simulink model "HaroldPractice"  (R2025b)
settings: Solver=VariableStepAuto  StartTime=0.0  StopTime=10.0  RelTol=1e-3
undefined symbols (not defined in the file): ChargingWire, DataIN, DataOUT, DisplayLink, OutputWire
settings Model: Creator=jakeo  LastModifiedBy=jakeo

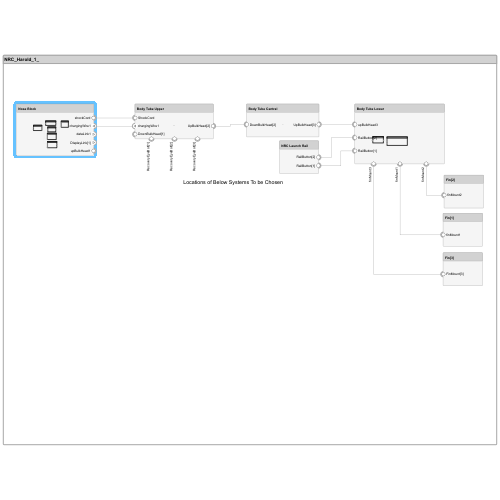
[thumbnail: Simulink's stored preview of the top-level diagram]
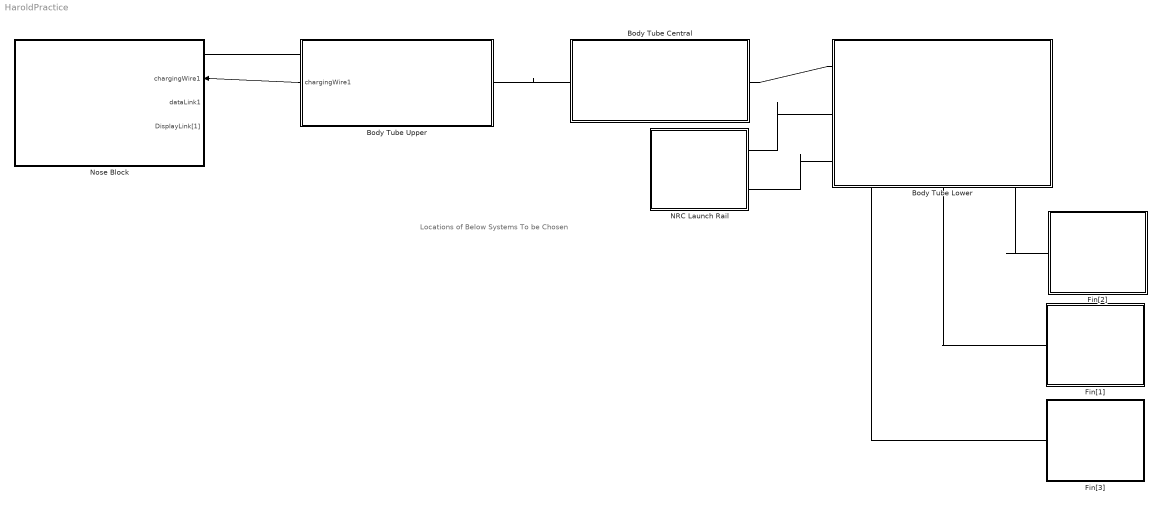
== system HaroldPractice ==
  note: Locations of Below Systems To be Chosen
  Body Tube Central : Subsystem
      settings: PortSchema="{\"entries\":[{\"content\":{\"headerSize\":26,\"margin\":15,\"minimumSpacing\":25,\"sides\":[{\"content\":{\"connectorIds\":[\"LConn1\"]},\"type\":\"ConnectorPlacement.EquallySpacedRectSide\",\"uuid\":\"03e957df-4bae-46ab-9d0d-48f80a496ac5\"},{\"content\":{\"connectorIds\":[\"RConn1\"],\"side\":\"RIGHT\"},\"type\":\"ConnectorPlacement.EquallySpacedRectSide\",\"uuid\":\"d2433d43-ba0e-4345-8a8e-99b57dcef125\"},{\"content\":{\"side\":\"TOP\"},\"type\":\"ConnectorPlacement.EquallySpacedRectSide\",\"uuid\":\"84844adf-0e3d-439c-a28c-7cf27e8d243a\"}]},\"type\":\"ConnectorPlacement.EquallySpacedConnector\",\"uuid\":\"9b26577b-50b2-4983-8f3c-4df87f23ba49\"}],\"packageUris\":[\"http://schema.mathworks.com/mf0/Connector/R2020b\"],\"version\":\"1.0\"}"
  Body Tube Lower : Subsystem
      settings: PortSchema="{\"entries\":[{\"content\":{\"headerSize\":26,\"margin\":15,\"minimumSpacing\":25,\"sides\":[{\"content\":{\"connectorIds\":[\"LConn1\",\"LConn4\",\"LConn5\"]},\"type\":\"ConnectorPlacement.EquallySpacedRectSide\",\"uuid\":\"03e957df-4bae-46ab-9d0d-48f80a496ac5\"},{\"content\":{\"side\":\"RIGHT\"},\"type\":\"ConnectorPlacement.EquallySpacedRectSide\",\"uuid\":\"d2433d43-ba0e-4345-8a8e-99b57dcef125\"},{\"content\":{\"side\":\"TOP\"},\"type\":\"ConnectorPlacement.EquallySpacedRectSide\",\"uuid\":\"84844adf-0e3d-439c-a28c-7cf27e8d243a\"},{\"content\":{\"connectorIds\":[\"LConn3\",\"LConn6\",\"LConn2\"],\"side\":\"BOTTOM\"},\"type\":\"ConnectorPlacement.EquallySpacedRectSide\",\"uuid\":\"9b3a5652-69bd-4b6e-9b29-131929afca7c\"}]},\"type\":\"ConnectorPlacement.EquallySpacedConnector\",\"uuid\":\"9b26577b-50b2-4983-8f3c-4df87f23ba49\"}],\"packageUris\":[\"http://schema.mathworks.com/mf0/Connector/R2020b\"],\"version\":\"1.0\"}"
  Body Tube Upper : Subsystem
      settings: PortSchema="{\"entries\":[{\"content\":{\"headerSize\":26,\"margin\":15,\"minimumSpacing\":25,\"sides\":[{\"content\":{\"connectorIds\":[\"LConn1\",\"Out1\",\"LConn2\"]},\"type\":\"ConnectorPlacement.EquallySpacedRectSide\",\"uuid\":\"03e957df-4bae-46ab-9d0d-48f80a496ac5\"},{\"content\":{\"connectorIds\":[\"RConn1\"],\"side\":\"RIGHT\"},\"type\":\"ConnectorPlacement.EquallySpacedRectSide\",\"uuid\":\"d2433d43-ba0e-4345-8a8e-99b57dcef125\"},{\"content\":{\"side\":\"TOP\"},\"type\":\"ConnectorPlacement.EquallySpacedRectSide\",\"uuid\":\"84844adf-0e3d-439c-a28c-7cf27e8d243a\"},{\"content\":{\"connectorIds\":[\"RConn2\",\"RConn3\",\"RConn4\"],\"side\":\"BOTTOM\"},\"type\":\"ConnectorPlacement.EquallySpacedRectSide\",\"uuid\":\"7d79bddd-aaf5-48a9-85da-385393746c36\"}]},\"type\":\"ConnectorPlacement.EquallySpacedConnector\",\"uuid\":\"9b26577b-50b2-4983-8f3c-4df87f23ba49\"}],\"packageUris\":[\"http://schema.mathworks.com/mf0/Connector/R2020b\"],\"version\":\"1.0\"}"
  Fin[1] : Subsystem
      settings: PortSchema="{\"entries\":[{\"content\":{\"headerSize\":26,\"margin\":15,\"minimumSpacing\":25,\"sides\":[{\"content\":{\"connectorIds\":[\"LConn1\"]},\"type\":\"ConnectorPlacement.EquallySpacedRectSide\",\"uuid\":\"03e957df-4bae-46ab-9d0d-48f80a496ac5\"},{\"content\":{\"side\":\"RIGHT\"},\"type\":\"ConnectorPlacement.EquallySpacedRectSide\",\"uuid\":\"d2433d43-ba0e-4345-8a8e-99b57dcef125\"},{\"content\":{\"side\":\"TOP\"},\"type\":\"ConnectorPlacement.EquallySpacedRectSide\",\"uuid\":\"84844adf-0e3d-439c-a28c-7cf27e8d243a\"}]},\"type\":\"ConnectorPlacement.EquallySpacedConnector\",\"uuid\":\"9b26577b-50b2-4983-8f3c-4df87f23ba49\"}],\"packageUris\":[\"http://schema.mathworks.com/mf0/Connector/R2020b\"],\"version\":\"1.0\"}"
  Fin[2] : Subsystem
      settings: PortSchema="{\"entries\":[{\"content\":{\"headerSize\":26,\"margin\":15,\"minimumSpacing\":25,\"sides\":[{\"content\":{\"connectorIds\":[\"LConn1\"]},\"type\":\"ConnectorPlacement.EquallySpacedRectSide\",\"uuid\":\"03e957df-4bae-46ab-9d0d-48f80a496ac5\"},{\"content\":{\"side\":\"RIGHT\"},\"type\":\"ConnectorPlacement.EquallySpacedRectSide\",\"uuid\":\"d2433d43-ba0e-4345-8a8e-99b57dcef125\"},{\"content\":{\"side\":\"TOP\"},\"type\":\"ConnectorPlacement.EquallySpacedRectSide\",\"uuid\":\"84844adf-0e3d-439c-a28c-7cf27e8d243a\"}]},\"type\":\"ConnectorPlacement.EquallySpacedConnector\",\"uuid\":\"9b26577b-50b2-4983-8f3c-4df87f23ba49\"}],\"packageUris\":[\"http://schema.mathworks.com/mf0/Connector/R2020b\"],\"version\":\"1.0\"}"
  Fin[3] : Subsystem
      settings: PortSchema="{\"entries\":[{\"content\":{\"headerSize\":26,\"margin\":15,\"minimumSpacing\":25,\"sides\":[{\"content\":{\"connectorIds\":[\"LConn1\"]},\"type\":\"ConnectorPlacement.EquallySpacedRectSide\",\"uuid\":\"03e957df-4bae-46ab-9d0d-48f80a496ac5\"},{\"content\":{\"side\":\"RIGHT\"},\"type\":\"ConnectorPlacement.EquallySpacedRectSide\",\"uuid\":\"d2433d43-ba0e-4345-8a8e-99b57dcef125\"},{\"content\":{\"side\":\"TOP\"},\"type\":\"ConnectorPlacement.EquallySpacedRectSide\",\"uuid\":\"84844adf-0e3d-439c-a28c-7cf27e8d243a\"}]},\"type\":\"ConnectorPlacement.EquallySpacedConnector\",\"uuid\":\"9b26577b-50b2-4983-8f3c-4df87f23ba49\"}],\"packageUris\":[\"http://schema.mathworks.com/mf0/Connector/R2020b\"],\"version\":\"1.0\"}"
  NRC Launch Rail : Subsystem
      settings: PortSchema="{\"entries\":[{\"content\":{\"headerSize\":26,\"margin\":15,\"minimumSpacing\":25,\"sides\":[{\"content\":{},\"type\":\"ConnectorPlacement.EquallySpacedRectSide\",\"uuid\":\"6f4db608-f49c-4d1a-85cc-b66ec62c2f96\"},{\"content\":{\"connectorIds\":[\"RConn2\",\"RConn1\"],\"side\":\"RIGHT\"},\"type\":\"ConnectorPlacement.EquallySpacedRectSide\",\"uuid\":\"3e275c67-1c5c-46cd-973f-75adcfca9e5d\"},{\"content\":{\"side\":\"TOP\"},\"type\":\"ConnectorPlacement.EquallySpacedRectSide\",\"uuid\":\"88fdcd36-c2bf-423f-a1bd-8e2b1c2ac438\"}]},\"type\":\"ConnectorPlacement.EquallySpacedConnector\",\"uuid\":\"596a3d77-8add-49e5-be48-e23e6a2b115a\"}],\"packageUris\":[\"http://schema.mathworks.com/mf0/Connector/R2020b\"],\"version\":\"1.0\"}"
  Nose Block : Subsystem
      settings: PortSchema="{\"entries\":[{\"content\":{\"headerSize\":26,\"margin\":15,\"minimumSpacing\":25,\"sides\":[{\"content\":{},\"type\":\"ConnectorPlacement.EquallySpacedRectSide\",\"uuid\":\"03e957df-4bae-46ab-9d0d-48f80a496ac5\"},{\"content\":{\"connectorIds\":[\"LConn1\",\"In1\",\"Out1\",\"Out2\",\"RConn1\"],\"side\":\"RIGHT\"},\"type\":\"ConnectorPlacement.EquallySpacedRectSide\",\"uuid\":\"d2433d43-ba0e-4345-8a8e-99b57dcef125\"},{\"content\":{\"side\":\"TOP\"},\"type\":\"ConnectorPlacement.EquallySpacedRectSide\",\"uuid\":\"84844adf-0e3d-439c-a28c-7cf27e8d243a\"}]},\"type\":\"ConnectorPlacement.EquallySpacedConnector\",\"uuid\":\"9b26577b-50b2-4983-8f3c-4df87f23ba49\"}],\"packageUris\":[\"http://schema.mathworks.com/mf0/Connector/R2020b\"],\"version\":\"1.0\"}"
  wires:
  Body Tube Upper/1(chargingWire1) -> Nose Block/1(chargingWire1)
  connections:
  Nose Block/LConn1 -- Body Tube Upper/LConn1
  Body Tube Upper/RConn1 -- Body Tube Central/LConn1
  Body Tube Central/RConn1 -- Body Tube Lower/LConn1
  Fin[2]/LConn1 -- Body Tube Lower/LConn2
  Fin[1]/LConn1 -- Body Tube Lower/LConn6
  Fin[3]/LConn1 -- Body Tube Lower/LConn3
  NRC Launch Rail/RConn1 -- Body Tube Lower/LConn5
  NRC Launch Rail/RConn2 -- Body Tube Lower/LConn4

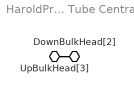
== system HaroldPractice/Body Tube Central ==
  DownBulkHead[2] : PMIOPort  Side=Left
  UpBulkHead[3] : PMIOPort  Port=2  Side=Right
  connections:
  UpBulkHead[3]/RConn1 -- DownBulkHead[2]/RConn1

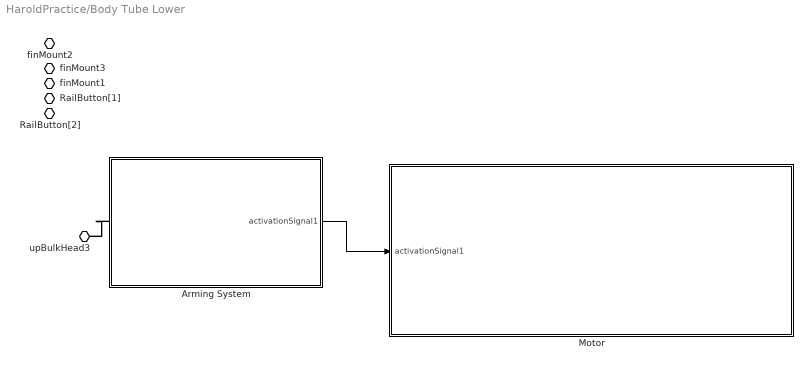
== system HaroldPractice/Body Tube Lower ==
  Arming System : Subsystem
      settings: PortSchema="{\"entries\":[{\"content\":{\"headerSize\":26,\"margin\":15,\"minimumSpacing\":25,\"sides\":[{\"content\":{\"connectorIds\":[\"LConn1\"]},\"type\":\"ConnectorPlacement.EquallySpacedRectSide\",\"uuid\":\"6f4db608-f49c-4d1a-85cc-b66ec62c2f96\"},{\"content\":{\"connectorIds\":[\"Out1\"],\"side\":\"RIGHT\"},\"type\":\"ConnectorPlacement.EquallySpacedRectSide\",\"uuid\":\"3e275c67-1c5c-46cd-973f-75adcfca9e5d\"},{\"content\":{\"side\":\"TOP\"},\"type\":\"ConnectorPlacement.EquallySpacedRectSide\",\"uuid\":\"88fdcd36-c2bf-423f-a1bd-8e2b1c2ac438\"}]},\"type\":\"ConnectorPlacement.EquallySpacedConnector\",\"uuid\":\"596a3d77-8add-49e5-be48-e23e6a2b115a\"}],\"packageUris\":[\"http://schema.mathworks.com/mf0/Connector/R2020b\"],\"version\":\"1.0\"}"
  Motor : Subsystem
      settings: PortSchema="{\"entries\":[{\"content\":{\"headerSize\":26,\"margin\":15,\"minimumSpacing\":25,\"sides\":[{\"content\":{\"connectorIds\":[\"LConn1\",\"In1\",\"LConn2\"]},\"type\":\"ConnectorPlacement.EquallySpacedRectSide\",\"uuid\":\"03e957df-4bae-46ab-9d0d-48f80a496ac5\"},{\"content\":{\"side\":\"RIGHT\"},\"type\":\"ConnectorPlacement.EquallySpacedRectSide\",\"uuid\":\"d2433d43-ba0e-4345-8a8e-99b57dcef125\"},{\"content\":{\"side\":\"TOP\"},\"type\":\"ConnectorPlacement.EquallySpacedRectSide\",\"uuid\":\"84844adf-0e3d-439c-a28c-7cf27e8d243a\"}]},\"type\":\"ConnectorPlacement.EquallySpacedConnector\",\"uuid\":\"9b26577b-50b2-4983-8f3c-4df87f23ba49\"}],\"packageUris\":[\"http://schema.mathworks.com/mf0/Connector/R2020b\"],\"version\":\"1.0\"}"
  upBulkHead3 : PMIOPort  Side=Left
  finMount2 : PMIOPort  Port=2  Side=Left
  finMount3 : PMIOPort  Port=3  Side=Left
  RailButton[2] : PMIOPort  Port=4  Side=Left
  RailButton[1] : PMIOPort  Port=5  Side=Left
  finMount1 : PMIOPort  Port=6  Side=Left
  wires:
  Arming System/1(activationSignal1) -> Motor/1(activationSignal1)
  connections:
  Arming System/LConn1 -- upBulkHead3/RConn1

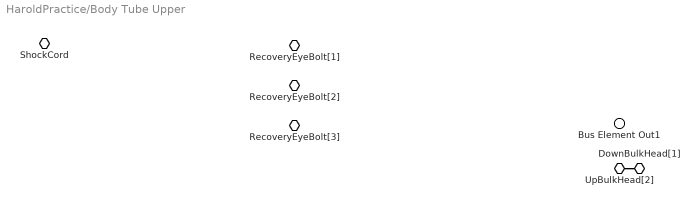
== system HaroldPractice/Body Tube Upper ==
  ShockCord : PMIOPort  Side=Left
  DownBulkHead[1] : PMIOPort  Port=2  Side=Left
  UpBulkHead[2] : PMIOPort  Port=3  Side=Right
  RecoveryEyeBolt[1] : PMIOPort  Port=4  Side=Right
  RecoveryEyeBolt[2] : PMIOPort  Port=5  Side=Right
  RecoveryEyeBolt[3] : PMIOPort  Port=6  Side=Right
  Bus Element Out1 : Outport  PortName=chargingWire1
  connections:
  UpBulkHead[2]/RConn1 -- DownBulkHead[1]/RConn1

== system HaroldPractice/Fin[1] ==
  finMount1 : PMIOPort  Side=Left

== system HaroldPractice/Fin[2] ==
  finMount2 : PMIOPort  Side=Left

== system HaroldPractice/Fin[3] ==
  FinMount[3] : PMIOPort  Side=Left

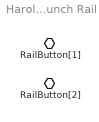
== system HaroldPractice/NRC Launch Rail ==
  RailButton[1] : PMIOPort  Side=Right
  RailButton[2] : PMIOPort  Port=2  Side=Right

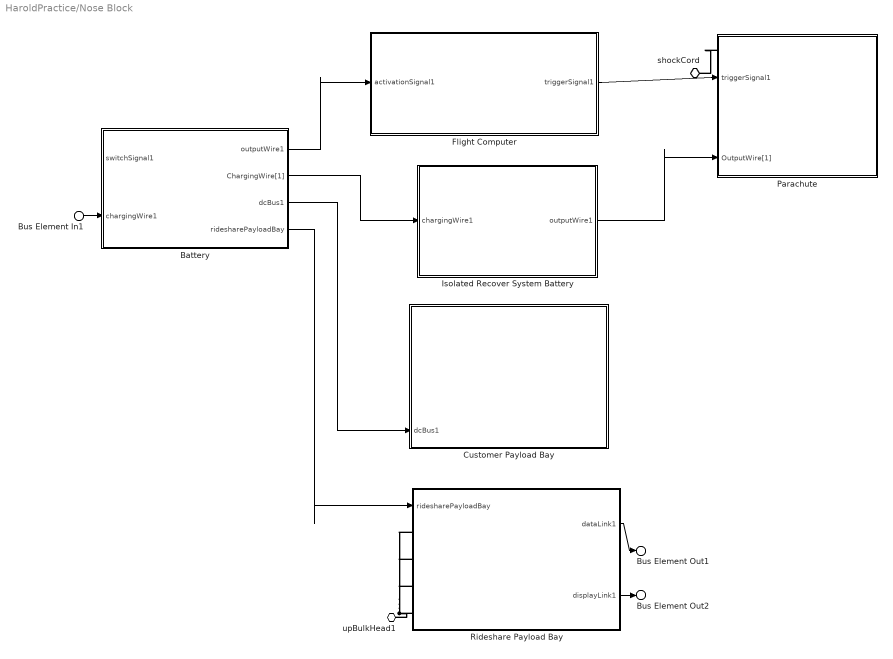
== system HaroldPractice/Nose Block ==
  Bus Element In1 : Inport  PortName=chargingWire1
  Battery : Subsystem
      settings: PortSchema="{\"entries\":[{\"content\":{\"headerSize\":26,\"margin\":15,\"minimumSpacing\":25,\"sides\":[{\"content\":{\"connectorIds\":[\"In1\",\"In2\"]},\"type\":\"ConnectorPlacement.EquallySpacedRectSide\",\"uuid\":\"03e957df-4bae-46ab-9d0d-48f80a496ac5\"},{\"content\":{\"connectorIds\":[\"Out1\",\"Out4\",\"Out2\",\"Out3\"],\"side\":\"RIGHT\"},\"type\":\"ConnectorPlacement.EquallySpacedRectSide\",\"uuid\":\"d2433d43-ba0e-4345-8a8e-99b57dcef125\"},{\"content\":{\"side\":\"TOP\"},\"type\":\"ConnectorPlacement.EquallySpacedRectSide\",\"uuid\":\"84844adf-0e3d-439c-a28c-7cf27e8d243a\"}]},\"type\":\"ConnectorPlacement.EquallySpacedConnector\",\"uuid\":\"9b26577b-50b2-4983-8f3c-4df87f23ba49\"}],\"packageUris\":[\"http://schema.mathworks.com/mf0/Connector/R2020b\"],\"version\":\"1.0\"}"
  Customer Payload Bay : Subsystem
      settings: PortSchema="{\"entries\":[{\"content\":{\"headerSize\":26,\"margin\":15,\"minimumSpacing\":25,\"sides\":[{\"content\":{\"connectorIds\":[\"LConn1\",\"LConn2\",\"LConn3\",\"LConn4\",\"In1\"]},\"type\":\"ConnectorPlacement.EquallySpacedRectSide\",\"uuid\":\"03e957df-4bae-46ab-9d0d-48f80a496ac5\"},{\"content\":{\"side\":\"RIGHT\"},\"type\":\"ConnectorPlacement.EquallySpacedRectSide\",\"uuid\":\"d2433d43-ba0e-4345-8a8e-99b57dcef125\"},{\"content\":{\"side\":\"TOP\"},\"type\":\"ConnectorPlacement.EquallySpacedRectSide\",\"uuid\":\"84844adf-0e3d-439c-a28c-7cf27e8d243a\"}]},\"type\":\"ConnectorPlacement.EquallySpacedConnector\",\"uuid\":\"9b26577b-50b2-4983-8f3c-4df87f23ba49\"}],\"packageUris\":[\"http://schema.mathworks.com/mf0/Connector/R2020b\"],\"version\":\"1.0\"}"
  Flight Computer : Subsystem
      settings: PortSchema="{\"entries\":[{\"content\":{\"headerSize\":26,\"margin\":15,\"minimumSpacing\":25,\"sides\":[{\"content\":{\"connectorIds\":[\"In1\"]},\"type\":\"ConnectorPlacement.EquallySpacedRectSide\",\"uuid\":\"6f4db608-f49c-4d1a-85cc-b66ec62c2f96\"},{\"content\":{\"connectorIds\":[\"Out1\"],\"side\":\"RIGHT\"},\"type\":\"ConnectorPlacement.EquallySpacedRectSide\",\"uuid\":\"3e275c67-1c5c-46cd-973f-75adcfca9e5d\"},{\"content\":{\"side\":\"TOP\"},\"type\":\"ConnectorPlacement.EquallySpacedRectSide\",\"uuid\":\"88fdcd36-c2bf-423f-a1bd-8e2b1c2ac438\"}]},\"type\":\"ConnectorPlacement.EquallySpacedConnector\",\"uuid\":\"596a3d77-8add-49e5-be48-e23e6a2b115a\"}],\"packageUris\":[\"http://schema.mathworks.com/mf0/Connector/R2020b\"],\"version\":\"1.0\"}"
  Isolated Recover System Battery : Subsystem
      settings: PortSchema="{\"entries\":[{\"content\":{\"headerSize\":26,\"margin\":15,\"minimumSpacing\":25,\"sides\":[{\"content\":{\"connectorIds\":[\"In1\"]},\"type\":\"ConnectorPlacement.EquallySpacedRectSide\",\"uuid\":\"6f4db608-f49c-4d1a-85cc-b66ec62c2f96\"},{\"content\":{\"connectorIds\":[\"Out1\"],\"side\":\"RIGHT\"},\"type\":\"ConnectorPlacement.EquallySpacedRectSide\",\"uuid\":\"3e275c67-1c5c-46cd-973f-75adcfca9e5d\"},{\"content\":{\"side\":\"TOP\"},\"type\":\"ConnectorPlacement.EquallySpacedRectSide\",\"uuid\":\"88fdcd36-c2bf-423f-a1bd-8e2b1c2ac438\"}]},\"type\":\"ConnectorPlacement.EquallySpacedConnector\",\"uuid\":\"596a3d77-8add-49e5-be48-e23e6a2b115a\"}],\"packageUris\":[\"http://schema.mathworks.com/mf0/Connector/R2020b\"],\"version\":\"1.0\"}"
  Parachute : Subsystem
      settings: PortSchema="{\"entries\":[{\"content\":{\"headerSize\":26,\"margin\":15,\"minimumSpacing\":25,\"sides\":[{\"content\":{\"connectorIds\":[\"LConn1\",\"In2\",\"LConn2\",\"LConn3\",\"In1\"]},\"type\":\"ConnectorPlacement.EquallySpacedRectSide\",\"uuid\":\"03e957df-4bae-46ab-9d0d-48f80a496ac5\"},{\"content\":{\"side\":\"RIGHT\"},\"type\":\"ConnectorPlacement.EquallySpacedRectSide\",\"uuid\":\"d2433d43-ba0e-4345-8a8e-99b57dcef125\"},{\"content\":{\"side\":\"TOP\"},\"type\":\"ConnectorPlacement.EquallySpacedRectSide\",\"uuid\":\"84844adf-0e3d-439c-a28c-7cf27e8d243a\"}]},\"type\":\"ConnectorPlacement.EquallySpacedConnector\",\"uuid\":\"9b26577b-50b2-4983-8f3c-4df87f23ba49\"}],\"packageUris\":[\"http://schema.mathworks.com/mf0/Connector/R2020b\"],\"version\":\"1.0\"}"
  Rideshare Payload Bay : Subsystem
      settings: PortSchema="{\"entries\":[{\"content\":{\"headerSize\":26,\"margin\":15,\"minimumSpacing\":25,\"sides\":[{\"content\":{\"connectorIds\":[\"In1\",\"LConn1\",\"LConn2\",\"LConn3\",\"LConn4\"]},\"type\":\"ConnectorPlacement.EquallySpacedRectSide\",\"uuid\":\"03e957df-4bae-46ab-9d0d-48f80a496ac5\"},{\"content\":{\"connectorIds\":[\"Out1\",\"Out2\"],\"side\":\"RIGHT\"},\"type\":\"ConnectorPlacement.EquallySpacedRectSide\",\"uuid\":\"d2433d43-ba0e-4345-8a8e-99b57dcef125\"},{\"content\":{\"side\":\"TOP\"},\"type\":\"ConnectorPlacement.EquallySpacedRectSide\",\"uuid\":\"84844adf-0e3d-439c-a28c-7cf27e8d243a\"}]},\"type\":\"ConnectorPlacement.EquallySpacedConnector\",\"uuid\":\"9b26577b-50b2-4983-8f3c-4df87f23ba49\"}],\"packageUris\":[\"http://schema.mathworks.com/mf0/Connector/R2020b\"],\"version\":\"1.0\"}"
  shockCord : PMIOPort  Side=Left
  upBulkHead1 : PMIOPort  Port=2  Side=Right
  Bus Element Out1 : Outport  PortName=dataLink1
  Bus Element Out2 : Outport  Port=2  PortName=DisplayLink[1]
  wires:
  Flight Computer/1(triggerSignal1) -> Parachute/2(triggerSignal1)
  Battery/1(outputWire1) -> Flight Computer/1(activationSignal1)
  Bus Element In1/1 -> Battery/2(chargingWire1)
  Rideshare Payload Bay/1(dataLink1) -> Bus Element Out1/1
  Rideshare Payload Bay/2(displayLink1) -> Bus Element Out2/1
  Battery/2(dcBus1) -> Customer Payload Bay/1(dcBus1)
  Battery/4(ChargingWire[1]) -> Isolated Recover System Battery/1(chargingWire1)
  Battery/3(ridesharePayloadBay) -> Rideshare Payload Bay/1(ridesharePayloadBay)
  Isolated Recover System Battery/1(outputWire1) -> Parachute/1(OutputWire[1])
  connections:
  Rideshare Payload Bay/LConn4 -- Rideshare Payload Bay/LConn1 -- Rideshare Payload Bay/LConn2 -- Rideshare Payload Bay/LConn3 -- upBulkHead1/RConn1
  Parachute/LConn1 -- shockCord/RConn1

== system HaroldPractice/Body Tube Lower/Arming System ==
  activation : PMIOPort  Side=Left
  Bus Element Out1 : Outport  PortName=activationSignal1

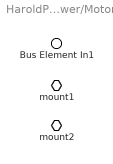
== system HaroldPractice/Body Tube Lower/Motor ==
  Bus Element In1 : Inport  PortName=activationSignal1
  mount1 : PMIOPort  Side=Left
  mount2 : PMIOPort  Port=2  Side=Left

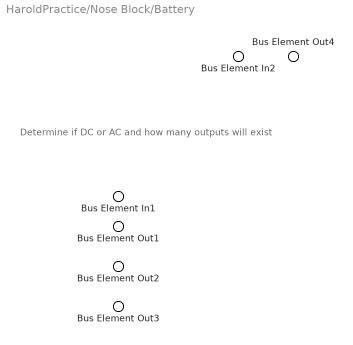
== system HaroldPractice/Nose Block/Battery ==
  note: Determine if DC or AC and how many outputs will exist
  Bus Element In2 : Inport  PortName=switchSignal1
  Bus Element In1 : Inport  Port=2  PortName=chargingWire1
  Bus Element Out1 : Outport  PortName=outputWire1
  Bus Element Out2 : Outport  Port=2  PortName=dcBus1
  Bus Element Out4 : Outport  Port=3  PortName=ridesharePayloadBay
  Bus Element Out3 : Outport  Port=4  PortName=ChargingWire[1]

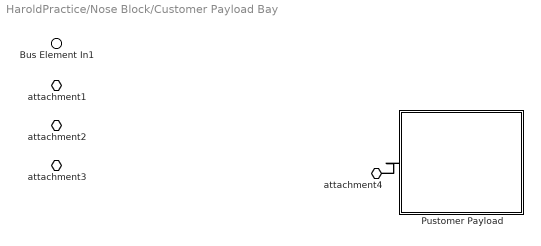
== system HaroldPractice/Nose Block/Customer Payload Bay ==
  Bus Element In1 : Inport  PortName=dcBus1
  Pustomer Payload : Subsystem
      settings: PortSchema="{\"entries\":[{\"content\":{\"headerSize\":26,\"margin\":15,\"minimumSpacing\":25,\"sides\":[{\"content\":{\"connectorIds\":[\"LConn1\"]},\"type\":\"ConnectorPlacement.EquallySpacedRectSide\",\"uuid\":\"03e957df-4bae-46ab-9d0d-48f80a496ac5\"},{\"content\":{\"side\":\"RIGHT\"},\"type\":\"ConnectorPlacement.EquallySpacedRectSide\",\"uuid\":\"d2433d43-ba0e-4345-8a8e-99b57dcef125\"},{\"content\":{\"side\":\"TOP\"},\"type\":\"ConnectorPlacement.EquallySpacedRectSide\",\"uuid\":\"84844adf-0e3d-439c-a28c-7cf27e8d243a\"}]},\"type\":\"ConnectorPlacement.EquallySpacedConnector\",\"uuid\":\"9b26577b-50b2-4983-8f3c-4df87f23ba49\"}],\"packageUris\":[\"http://schema.mathworks.com/mf0/Connector/R2020b\"],\"version\":\"1.0\"}"
  attachment1 : PMIOPort  Side=Left
  attachment2 : PMIOPort  Port=2  Side=Left
  attachment3 : PMIOPort  Port=3  Side=Left
  attachment4 : PMIOPort  Port=4  Side=Left
  connections:
  Pustomer Payload/LConn1 -- attachment4/RConn1

== system HaroldPractice/Nose Block/Flight Computer ==
  Bus Element In1 : Inport  PortName=activationSignal1
  Bus Element Out1 : Outport  PortName=triggerSignal1

== system HaroldPractice/Nose Block/Isolated Recover System Battery ==
  Bus Element In1 : Inport  PortName=chargingWire1
  Bus Element Out1 : Outport  PortName=outputWire1

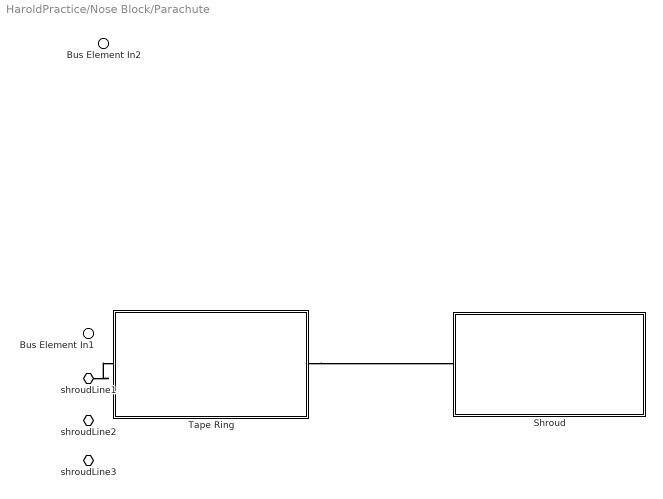
== system HaroldPractice/Nose Block/Parachute ==
  Bus Element In2 : Inport  PortName=OutputWire[1]
  Bus Element In1 : Inport  Port=2  PortName=triggerSignal1
  Shroud : Subsystem
      settings: PortSchema="{\"entries\":[{\"content\":{\"headerSize\":26,\"margin\":15,\"minimumSpacing\":25,\"sides\":[{\"content\":{\"connectorIds\":[\"LConn1\"]},\"type\":\"ConnectorPlacement.EquallySpacedRectSide\",\"uuid\":\"03e957df-4bae-46ab-9d0d-48f80a496ac5\"},{\"content\":{\"side\":\"RIGHT\"},\"type\":\"ConnectorPlacement.EquallySpacedRectSide\",\"uuid\":\"d2433d43-ba0e-4345-8a8e-99b57dcef125\"},{\"content\":{\"side\":\"TOP\"},\"type\":\"ConnectorPlacement.EquallySpacedRectSide\",\"uuid\":\"84844adf-0e3d-439c-a28c-7cf27e8d243a\"}]},\"type\":\"ConnectorPlacement.EquallySpacedConnector\",\"uuid\":\"9b26577b-50b2-4983-8f3c-4df87f23ba49\"}],\"packageUris\":[\"http://schema.mathworks.com/mf0/Connector/R2020b\"],\"version\":\"1.0\"}"
  Tape Ring : Subsystem
      settings: PortSchema="{\"entries\":[{\"content\":{\"headerSize\":26,\"margin\":15,\"minimumSpacing\":25,\"sides\":[{\"content\":{\"connectorIds\":[\"LConn1\"]},\"type\":\"ConnectorPlacement.EquallySpacedRectSide\",\"uuid\":\"03e957df-4bae-46ab-9d0d-48f80a496ac5\"},{\"content\":{\"connectorIds\":[\"RConn1\"],\"side\":\"RIGHT\"},\"type\":\"ConnectorPlacement.EquallySpacedRectSide\",\"uuid\":\"d2433d43-ba0e-4345-8a8e-99b57dcef125\"},{\"content\":{\"side\":\"TOP\"},\"type\":\"ConnectorPlacement.EquallySpacedRectSide\",\"uuid\":\"84844adf-0e3d-439c-a28c-7cf27e8d243a\"}]},\"type\":\"ConnectorPlacement.EquallySpacedConnector\",\"uuid\":\"9b26577b-50b2-4983-8f3c-4df87f23ba49\"}],\"packageUris\":[\"http://schema.mathworks.com/mf0/Connector/R2020b\"],\"version\":\"1.0\"}"
  shroudLine1 : PMIOPort  Side=Left
  shroudLine2 : PMIOPort  Port=2  Side=Left
  shroudLine3 : PMIOPort  Port=3  Side=Left
  connections:
  shroudLine1/RConn1 -- Tape Ring/LConn1
  Tape Ring/RConn1 -- Shroud/LConn1

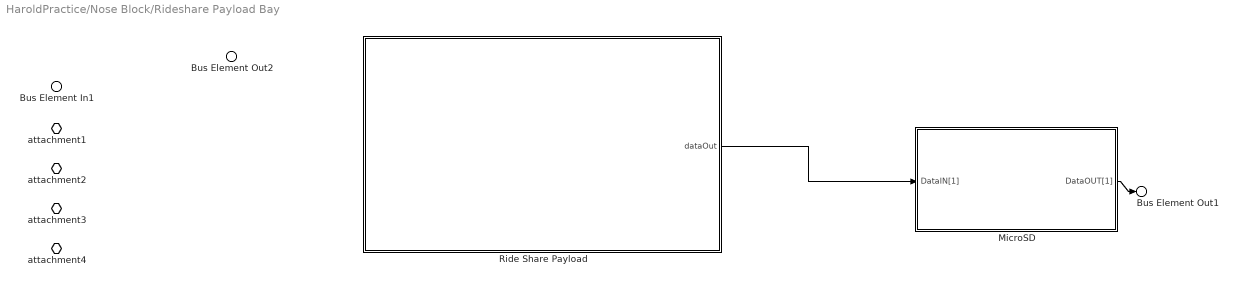
== system HaroldPractice/Nose Block/Rideshare Payload Bay ==
  Bus Element In1 : Inport  PortName=ridesharePayloadBay
  MicroSD : Subsystem
      settings: PortSchema="{\"entries\":[{\"content\":{\"headerSize\":26,\"margin\":15,\"minimumSpacing\":25,\"sides\":[{\"content\":{\"connectorIds\":[\"In1\"]},\"type\":\"ConnectorPlacement.EquallySpacedRectSide\",\"uuid\":\"6f4db608-f49c-4d1a-85cc-b66ec62c2f96\"},{\"content\":{\"connectorIds\":[\"Out1\"],\"side\":\"RIGHT\"},\"type\":\"ConnectorPlacement.EquallySpacedRectSide\",\"uuid\":\"3e275c67-1c5c-46cd-973f-75adcfca9e5d\"},{\"content\":{\"side\":\"TOP\"},\"type\":\"ConnectorPlacement.EquallySpacedRectSide\",\"uuid\":\"88fdcd36-c2bf-423f-a1bd-8e2b1c2ac438\"}]},\"type\":\"ConnectorPlacement.EquallySpacedConnector\",\"uuid\":\"596a3d77-8add-49e5-be48-e23e6a2b115a\"}],\"packageUris\":[\"http://schema.mathworks.com/mf0/Connector/R2020b\"],\"version\":\"1.0\"}"
  Ride Share Payload : Subsystem
      settings: PortSchema="{\"entries\":[{\"content\":{\"headerSize\":26,\"margin\":15,\"minimumSpacing\":25,\"sides\":[{\"content\":{},\"type\":\"ConnectorPlacement.EquallySpacedRectSide\",\"uuid\":\"03e957df-4bae-46ab-9d0d-48f80a496ac5\"},{\"content\":{\"connectorIds\":[\"Out1\"],\"side\":\"RIGHT\"},\"type\":\"ConnectorPlacement.EquallySpacedRectSide\",\"uuid\":\"d2433d43-ba0e-4345-8a8e-99b57dcef125\"},{\"content\":{\"side\":\"TOP\"},\"type\":\"ConnectorPlacement.EquallySpacedRectSide\",\"uuid\":\"84844adf-0e3d-439c-a28c-7cf27e8d243a\"}]},\"type\":\"ConnectorPlacement.EquallySpacedConnector\",\"uuid\":\"9b26577b-50b2-4983-8f3c-4df87f23ba49\"}],\"packageUris\":[\"http://schema.mathworks.com/mf0/Connector/R2020b\"],\"version\":\"1.0\"}"
  attachment1 : PMIOPort  Side=Left
  attachment2 : PMIOPort  Port=2  Side=Left
  attachment3 : PMIOPort  Port=3  Side=Left
  attachment4 : PMIOPort  Port=4  Side=Left
  Bus Element Out1 : Outport  PortName=dataLink1
  Bus Element Out2 : Outport  Port=2  PortName=displayLink1
  wires:
  Ride Share Payload/1(dataOut) -> MicroSD/1(DataIN[1])
  MicroSD/1(DataOUT[1]) -> Bus Element Out1/1

== system HaroldPractice/Nose Block/Customer Payload Bay/Pustomer Payload ==
  DCBus[1] : PMIOPort  Side=Left

== system HaroldPractice/Nose Block/Parachute/Shroud ==
  shroudLines2 : PMIOPort  Side=Left

== system HaroldPractice/Nose Block/Parachute/Tape Ring ==
  shroudLines1 : PMIOPort  Side=Left
  shroudLines2 : PMIOPort  Port=2  Side=Right

== system HaroldPractice/Nose Block/Rideshare Payload Bay/MicroSD ==
  Bus Element In1 : Inport  PortName=DataIN[1]
  Bus Element Out1 : Outport  PortName=DataOUT[1]

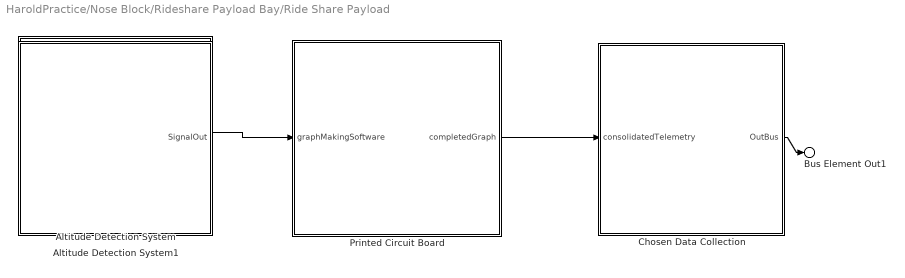
== system HaroldPractice/Nose Block/Rideshare Payload Bay/Ride Share Payload ==
  Altitude Detection System : Subsystem
      settings: PortSchema="{\"entries\":[{\"content\":{\"headerSize\":26,\"margin\":15,\"minimumSpacing\":25,\"sides\":[{\"content\":{},\"type\":\"ConnectorPlacement.EquallySpacedRectSide\",\"uuid\":\"6f4db608-f49c-4d1a-85cc-b66ec62c2f96\"},{\"content\":{\"connectorIds\":[\"Out1\"],\"side\":\"RIGHT\"},\"type\":\"ConnectorPlacement.EquallySpacedRectSide\",\"uuid\":\"3e275c67-1c5c-46cd-973f-75adcfca9e5d\"},{\"content\":{\"side\":\"TOP\"},\"type\":\"ConnectorPlacement.EquallySpacedRectSide\",\"uuid\":\"88fdcd36-c2bf-423f-a1bd-8e2b1c2ac438\"}]},\"type\":\"ConnectorPlacement.EquallySpacedConnector\",\"uuid\":\"596a3d77-8add-49e5-be48-e23e6a2b115a\"}],\"packageUris\":[\"http://schema.mathworks.com/mf0/Connector/R2020b\"],\"version\":\"1.0\"}"
  Altitude Detection System1 : Subsystem
      settings: PortSchema="{\"entries\":[{\"content\":{\"headerSize\":26,\"margin\":15,\"minimumSpacing\":25,\"sides\":[{\"content\":{},\"type\":\"ConnectorPlacement.EquallySpacedRectSide\",\"uuid\":\"6f4db608-f49c-4d1a-85cc-b66ec62c2f96\"},{\"content\":{\"connectorIds\":[\"Out1\"],\"side\":\"RIGHT\"},\"type\":\"ConnectorPlacement.EquallySpacedRectSide\",\"uuid\":\"3e275c67-1c5c-46cd-973f-75adcfca9e5d\"},{\"content\":{\"side\":\"TOP\"},\"type\":\"ConnectorPlacement.EquallySpacedRectSide\",\"uuid\":\"88fdcd36-c2bf-423f-a1bd-8e2b1c2ac438\"}]},\"type\":\"ConnectorPlacement.EquallySpacedConnector\",\"uuid\":\"596a3d77-8add-49e5-be48-e23e6a2b115a\"}],\"packageUris\":[\"http://schema.mathworks.com/mf0/Connector/R2020b\"],\"version\":\"1.0\"}"
  Chosen Data Collection : Subsystem
      settings: PortSchema="{\"entries\":[{\"content\":{\"headerSize\":26,\"margin\":15,\"minimumSpacing\":25,\"sides\":[{\"content\":{\"connectorIds\":[\"In1\"]},\"type\":\"ConnectorPlacement.EquallySpacedRectSide\",\"uuid\":\"6f4db608-f49c-4d1a-85cc-b66ec62c2f96\"},{\"content\":{\"connectorIds\":[\"Out1\"],\"side\":\"RIGHT\"},\"type\":\"ConnectorPlacement.EquallySpacedRectSide\",\"uuid\":\"3e275c67-1c5c-46cd-973f-75adcfca9e5d\"},{\"content\":{\"side\":\"TOP\"},\"type\":\"ConnectorPlacement.EquallySpacedRectSide\",\"uuid\":\"88fdcd36-c2bf-423f-a1bd-8e2b1c2ac438\"}]},\"type\":\"ConnectorPlacement.EquallySpacedConnector\",\"uuid\":\"596a3d77-8add-49e5-be48-e23e6a2b115a\"}],\"packageUris\":[\"http://schema.mathworks.com/mf0/Connector/R2020b\"],\"version\":\"1.0\"}"
  Printed Circuit Board : Subsystem
      settings: PortSchema="{\"entries\":[{\"content\":{\"headerSize\":26,\"margin\":15,\"minimumSpacing\":25,\"sides\":[{\"content\":{\"connectorIds\":[\"In1\"]},\"type\":\"ConnectorPlacement.EquallySpacedRectSide\",\"uuid\":\"6f4db608-f49c-4d1a-85cc-b66ec62c2f96\"},{\"content\":{\"connectorIds\":[\"Out1\"],\"side\":\"RIGHT\"},\"type\":\"ConnectorPlacement.EquallySpacedRectSide\",\"uuid\":\"3e275c67-1c5c-46cd-973f-75adcfca9e5d\"},{\"content\":{\"side\":\"TOP\"},\"type\":\"ConnectorPlacement.EquallySpacedRectSide\",\"uuid\":\"88fdcd36-c2bf-423f-a1bd-8e2b1c2ac438\"}]},\"type\":\"ConnectorPlacement.EquallySpacedConnector\",\"uuid\":\"596a3d77-8add-49e5-be48-e23e6a2b115a\"}],\"packageUris\":[\"http://schema.mathworks.com/mf0/Connector/R2020b\"],\"version\":\"1.0\"}"
  Bus Element Out1 : Outport  PortName=dataOut
  wires:
  Altitude Detection System/1(Graph making software) -> Printed Circuit Board/1(graphMakingSoftware)
  Printed Circuit Board/1(completedGraph) -> Chosen Data Collection/1(consolidatedTelemetry)
  Chosen Data Collection/1(OutBus) -> Bus Element Out1/1

== system HaroldPractice/Nose Block/Rideshare Payload Bay/Ride Share Payload/Altitude Detection System ==
  Bus Element Out1 : Outport  PortName=Graph making software

== system HaroldPractice/Nose Block/Rideshare Payload Bay/Ride Share Payload/Altitude Detection System1 ==
  Bus Element Out1 : Outport  PortName=SignalOut

== system HaroldPractice/Nose Block/Rideshare Payload Bay/Ride Share Payload/Chosen Data Collection ==
  Bus Element In1 : Inport  PortName=consolidatedTelemetry
  Bus Element Out1 : Outport  PortName=OutBus

== system HaroldPractice/Nose Block/Rideshare Payload Bay/Ride Share Payload/Printed Circuit Board ==
  Bus Element In1 : Inport  PortName=graphMakingSoftware
  Bus Element Out1 : Outport  PortName=completedGraph
